simulink model "L22B1"  (R2015a)
settings: Solver=ode45  StartTime=0.0  StopTime=1  MaxStep=1e-4  RelTol=1e-3
values from neighbouring files (symbols this model uses):
  a1 = ke*km/J/La    (= 10740.9160847)    [L22m.m]
  a2 = Ra/La    (= 294.117647059)    [L22m.m]
  alfaConstant = 1.31    [L22m.m]
  b = -km*kp/J/La    (= -1139188.06959)    [L22m.m]
  cB1 = 290    [L22m.m]
  fmaxB1 = 1e+7    (= 10000000)    [L22m.m]
  J = 0.71e-3    (= 0.00071)    [L22m.m]
  ke = 0.33    [L22m.m]
  km = ke    (= 0.33)    [L22m.m]
  kp = 35    [L22m.m]
  La = 14.28e-3    (= 0.01428)    [L22m.m]
  Ra = 4.2    [L22m.m]
  TiB1 = 0.0234    [L22m.m]
  v = -12    [L22m.m]
  vTime = 0.6    [L22m.m]
  w = 20    [L22m.m]
settings Model: Creator=B014-5  LastModifiedBy=B014-5

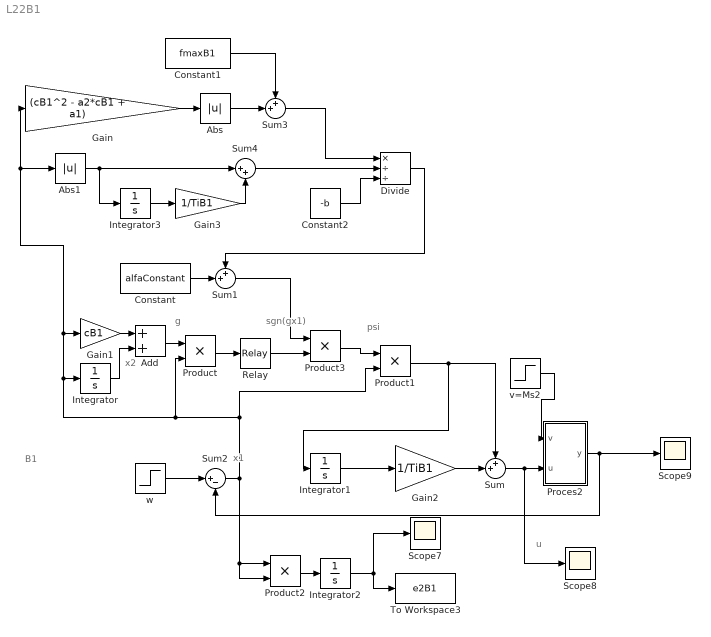
== system L22B1 ==
  note: u
  note: psi
  note: g
  note: sgn(gx1)
  note: x2
  note: x1
  note: B1
  Abs : Abs
  Abs1 : Abs
  Add : Sum
  Constant : Constant  Value=alfaConstant
  Constant1 : Constant  Value=fmaxB1
  Constant2 : Constant  Value=-b
  Divide : Product  Inputs=*//
  Gain : Gain  Gain=(cB1^2 - a2*cB1 + a1)
  Gain1 : Gain  Gain=cB1
  Gain2 : Gain  Gain=1/TiB1
  Gain3 : Gain  Gain=1/TiB1
  Integrator{,1..3} (4 alike) : Integrator
  Proces2 : Subsystem
  Product{,1..3} (4 alike) : Product
  Relay : Relay  OnSwitchValue=0  OffSwitchValue=0  OffOutputValue=-1  ZeroCross=off
  Scope7 : Scope
      settings: SaveName=ScopeData8
  Scope8 : Scope
      settings: YMin=-4.25e+105  YMax=0  SaveName=ScopeData10
  Scope9 : Scope
      settings: YMin=-4.25e+105  YMax=0  SaveName=ScopeData6
  Sum : Sum  Inputs=++|
  Sum1 : Sum  Inputs=++|
  Sum2 : Sum  Inputs=|+-
  Sum3 : Sum  Inputs=++|
  Sum4 : Sum  Inputs=|++
  To Workspace3 : ToWorkspace  VariableName=e2B1  SampleTime=-1
  v=Ms2 : Step  Time=vTime  After=v  SampleTime=0
  w : Step  Time=0  After=w  SampleTime=0
  wires:
  w/1 -> Sum2/1
  Proces2/1(y) -> Scope9/1, Sum2/2
  Product1/1 -> Integrator1/1, Sum/1
  Sum/1 -> Scope8/1, Proces2/2(u)
  Relay/1 -> Product3/2
  Sum2/1 -> Integrator/1, Gain/1, Abs1/1, Gain1/1, Product/2, Product1/2, Product2/1, Product2/2
  Gain1/1 -> Add/1
  Integrator/1 -> Add/2
  Product/1 -> Relay/1
  Add/1 -> Product/1
  Product3/1 -> Product1/1
  Integrator1/1 -> Gain2/1
  Gain2/1 -> Sum/2
  v=Ms2/1 -> Proces2/1(v)
  Product2/1 -> Integrator2/1
  Integrator2/1 -> Scope7/1, To Workspace3/1
  Sum1/1 -> Product3/1
  Constant/1 -> Sum1/2
  Gain/1 -> Abs/1
  Abs/1 -> Sum3/2
  Constant1/1 -> Sum3/1
  Sum3/1 -> Divide/1
  Abs1/1 -> Integrator3/1, Sum4/1
  Integrator3/1 -> Gain3/1
  Gain3/1 -> Sum4/2
  Sum4/1 -> Divide/2
  Divide/1 -> Sum1/1
  Constant2/1 -> Divide/3

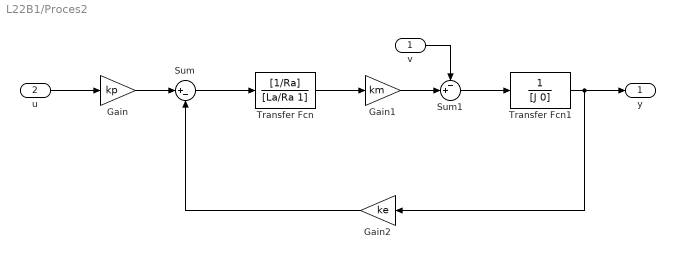
== system L22B1/Proces2 ==
  v : Inport
  u : Inport  Port=2
  Gain : Gain  Gain=kp
  Gain1 : Gain  Gain=km
  Gain2 : Gain  Gain=ke
  Sum : Sum  Inputs=|+-
  Sum1 : Sum  Inputs=-+|
  Transfer Fcn : TransferFcn  Numerator=[1/Ra]  Denominator=[La/Ra 1]
  Transfer Fcn1 : TransferFcn  Denominator=[J 0]
  y : Outport
  wires:
  Transfer Fcn/1 -> Gain1/1
  Gain1/1 -> Sum1/2
  u/1 -> Gain/1
  Gain2/1 -> Sum/2
  Sum/1 -> Transfer Fcn/1
  Sum1/1 -> Transfer Fcn1/1
  Transfer Fcn1/1 -> Gain2/1, y/1
  Gain/1 -> Sum/1
  v/1 -> Sum1/1
